simulink model "ControlPenduloInvertidoLineal"  (R2024b)
settings: Solver=VariableStepAuto  StartTime=0.0  StopTime=50  RelTol=1e-3
libraries: fuzblock x1
settings Model: Creator=user  LastModifiedBy=user

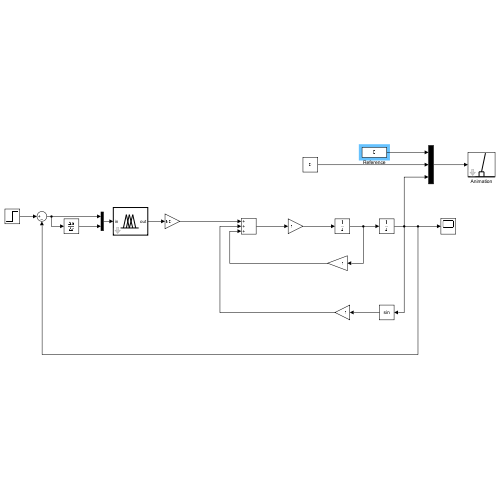
[thumbnail: Simulink's stored preview of the top-level diagram]
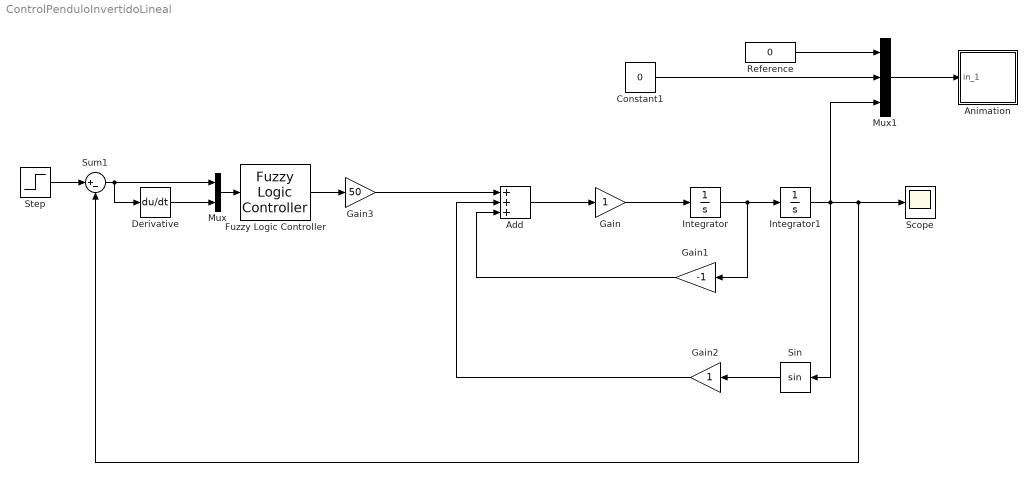
== system ControlPenduloInvertidoLineal ==
  Add : Sum  Inputs=+++
  Animation : Subsystem  mask(Pendulum plot){RefBlock=Reference}
      mask prompts: RefBlock "DC reference signal block name:"
      mask help: Pendulum plot
      mask Help: Pendulum animation function using Handle graphics.
      mask Display: plot([-10 10],[0 0],[-2 -2 2 2],[0 1 1 0],[0 3],[1 5])
  Constant1 : Constant  Value=0
  Derivative : Derivative
  Fuzzy Logic Controller : fuzblock/Fuzzy Logic  Controller  FIS='LogicaPendulo.fis'  OutputSampleNumber=101  DataType=double  FuzzifiedInputs=off  RuleFiringStrengths=off  RuleOutputs=off  AggregatedOutputs=off  SimulateUsing=Interpreted execution  OutOfRangeInputValueMessage=warning  NoRuleFiredMessage=warning  EmptyOutputFuzzySetMessage=warning
  Gain : Gain
  Gain1 : Gain  Gain=-1
  Gain2 : Gain
  Gain3 : Gain  Gain=50
  Integrator : Integrator
  Integrator1 : Integrator  InitialCondition=2
  Mux : Mux  Inputs=2
  Mux1 : Mux  Inputs=3
  Reference : Constant  Value=0
  Scope : Scope
  Sin : Trigonometry
  Step : Step  After=0  SampleTime=0
  Sum1 : Sum  Inputs=|+-
  wires:
  Add/1 -> Gain/1
  Gain/1 -> Integrator/1
  Integrator/1 -> Gain1/1, Integrator1/1
  Gain1/1 -> Add/3
  Gain2/1 -> Add/2
  Sin/1 -> Gain2/1
  Step/1 -> Sum1/1
  Derivative/1 -> Mux/2
  Sum1/1 -> Derivative/1, Mux/1
  Mux/1 -> Fuzzy Logic Controller/1
  Gain3/1 -> Add/1
  Fuzzy Logic Controller/1 -> Gain3/1
  Integrator1/1 -> Sin/1, Scope/1, Sum1/2, Mux1/3
  Reference/1 -> Mux1/1
  Constant1/1 -> Mux1/2
  Mux1/1 -> Animation/1(in_1)

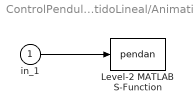
== system ControlPenduloInvertidoLineal/Animation ==
  in_1 : Inport
  Level-2 MATLAB S-Function : M-S-Function  FunctionName=pendan  Parameters=RefBlock
  wires:
  in_1/1 -> Level-2 MATLAB S-Function/1
